simulink model "motor_ctl_sm"  (R2023a)
settings: configuration reference "config" (kept outside this file)
model workspace (MAT data in the model file):
  enc_line_inv_p_n = Simulink.Parameter
  enc_line_inv_p_n.Value = 0.0001
  enc_line_inv_p_n.Description = '编码器分辨率 倒数   
    | '
  enc_line_inv_p_n.DataType = 'single'
  enc_line_inv_p_n.Complexity = 'real'
  enc_line_inv_p_n.Dimensions = [1 1]
  init_flag = Simulink.Signal
  init_flag.Description = '初始化信号  0  1 需要被初始化'
  init_flag.DataType = 'uint8'
  init_flag.Dimensions = 1
  init_flag.DimensionsMode = 'auto'
  init_flag.Complexity = 'auto'
  init_flag.SampleTime = -1
  init_flag.SamplingMode = 'auto'
  kFs = Simulink.Parameter
  kFs.Value = 10000
  kFs.Description = '位置环 速度环执行频率  仅用于仿真'
  kFs.DataType = 'double'
  kFs.Complexity = 'real'
  kFs.Dimensions = [1 1]
  tp = Simulink.Parameter
  tp.Value = 0.0001
  tp.Description = '位置环速度环执行周期  s'
  tp.DataType = 'single'
  tp.Complexity = 'real'
  tp.Dimensions = [1 1]
  wn_Hz = Simulink.Parameter
  wn_Hz.Value = 400
  wn_Hz.Description = '速度观测器带宽 Hz'
  wn_Hz.DataType = 'single'
  wn_Hz.Complexity = 'real'
  wn_Hz.Dimensions = [1 1]
settings Model: DataDictionary=model_config.sldd  ParameterArgumentNames=enc_line_inv_p_n,tp,wn_Hz  Creator=huangcheng  LastModifiedBy=Administrator
settings ConfigSetRef: SourceName=config

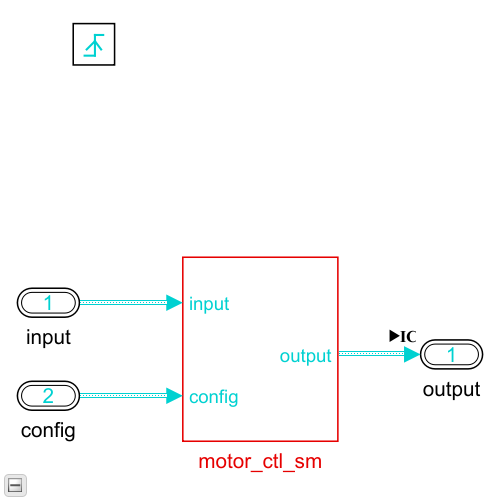
[thumbnail: Simulink's stored preview of the top-level diagram]
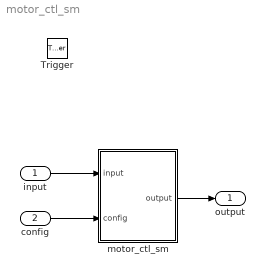
== system motor_ctl_sm ==
  input : Inport  OutDataTypeStr=Bus: MotorCtlSmInput  BusOutputAsStruct=on
  config : Inport  Port=2  OutDataTypeStr=Bus: MotorCtlSmConfig  BusOutputAsStruct=on
  Trigger : TriggerPort  VariantControl=(inherit)  PortDimensions=1
  motor_ctl_sm : Subsystem
  output : Outport  OutDataTypeStr=Bus: MotorCtlSmOutput  BusOutputAsStruct=on
  wires:
  input/1 -> motor_ctl_sm/1(input)
  config/1 -> motor_ctl_sm/2(config)
  motor_ctl_sm/1(output) -> output/1

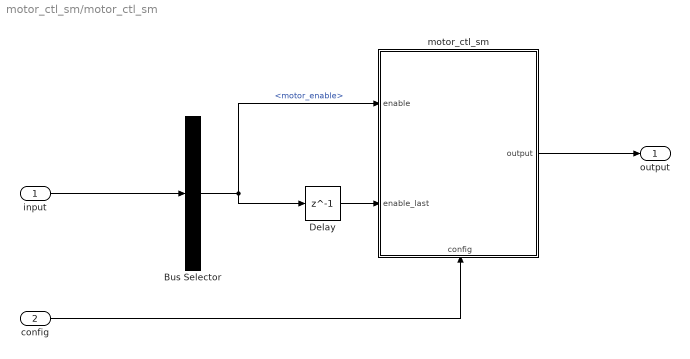
== system motor_ctl_sm/motor_ctl_sm ==
  input : Inport  OutDataTypeStr=Bus: MotorCtlSmInput
  config : Inport  Port=2  OutDataTypeStr=Bus: MotorCtlSmConfig
  Bus Selector : BusSelector  OutputSignals=motor_enable
  Delay : Delay  DelayLength=1  StateName=motor_enable_last
  motor_ctl_sm : Stateflow chart
      settings: RTWSystemCode=Reusable function  PortSchema="{\"entries\":[{\"content\":{\"sides\":[{\"content\":{\"connectorIds\":[\"In2\",\"In3\"]},\"type\":\"ConnectorPlacement.EquallySpacedRectSide\",\"uuid\":\"4756ae5c-8ae8-4bde-9ee8-e3b772b98f84\"},{\"content\":{\"connectorIds\":[\"Out1\"],\"side\":\"RIGHT\"},\"type\":\"ConnectorPlacement.EquallySpacedRectSide\",\"uuid\":\"1f9a028f-a8f7-4623-98a8-242534b898db\"},{\"content\":{\"side\":\"TOP\"},\"type\":\"ConnectorPlacement.EquallySpacedRectSide\",\"uuid\":\"fc85aa74-54fe-41b6-9575-751a8728c497\"},{\"content\":{\"connectorIds\":[\"In1\"],\"side\":\"BOTTOM\"},\"type\":\"ConnectorPlacement.EquallySpacedRectSide\",\"uuid\":\"2f151dbf-d119-42f2-9ccc-419d1265f28c\"}]},\"type\":\"ConnectorPlacement.EquallySpacedConnector\",\"uuid\":\"14a80403-31f4-4019-911b-7e14be7a3597\"}],\"packageUris\":[\"http://schema.mathworks.com/mf0/Connector/R2020b\"],\"version\":\"1.0\"}"
  output : Outport
  wires:
  Delay/1 -> motor_ctl_sm/3(enable_last)
  Bus Selector/1 -> motor_ctl_sm/2(enable), Delay/1  "<motor_enable>"
  motor_ctl_sm/1(output) -> output/1
  input/1 -> Bus Selector/1
  config/1 -> motor_ctl_sm/1(config)

== stateflow chart motor_ctl_sm/motor_ctl_sm ==
  state disable
    du:
    output.state = 0;
    output.error = 0;
    output.warning = 0;
    output.mode_now = config.mode;
  state enable
    en:
    output.state = 1;
    du:
    output.error = 0;
    output.warning = 0;
    output.mode_now = config.mode;
  state error
    du:
    output.state = -1;
    output.error = 0;
    output.warning = 0;
    output.mode_now =  config.mode;
  (default) -> disable
  enable -> disable [order 2] : [enable == 0]
  disable -> enable [order 2] : [enable_last == 0 && enable == 1]
  disable -> error [order 1] : [output.error ~= 0]
  error -> disable : [enable_last == 0 && enable == 3]
  enable -> error [order 1] : [output.error ~= 0]
  data: config input Bus: MotorCtlSmConfig; enable input; enable_last input; output output Bus: MotorCtlSmOutput
